simulink model "linear_exp_2025a"  (R2025a)
settings: Solver=FixedStepDiscrete  StartTime=0.0  StopTime=Inf  FixedStep=Ts  RelTol=1e-3
model workspace (MAT data in the model file):
  p_active = Simulink.Parameter
  p_active.Value = 1
  p_active.Complexity = 'real'
  p_active.Dimensions = [1 1]
  p_active.DataType = 'auto'
  p_ff = Simulink.Parameter
  p_ff.Value = [-1.41559534854 -1.58206727697 -1.65093789551 -1.60998265668 -1.49289778237 -1.36268185504 -1.28204754292 -1.28521947357 -1.3635848216 -1.47038204607 -1.54100339838 -1.51955701219 ... (800000 elements, 1x800000)]
  p_ff.Complexity = 'real'
  p_ff.Dimensions = [1 800000]
  p_ff.DataType = 'auto'
  p_ref = Simulink.Parameter
  p_ref.Value = [0 0 0 0 0 0 0 0 0 0 0 0 ... (800000 elements, 800000x1)]
  p_ref.Complexity = 'real'
  p_ref.Dimensions = [800000 1]
  p_ref.DataType = 'auto'
  p_servo = Simulink.Parameter
  p_servo.Value = 0
  p_servo.Complexity = 'real'
  p_servo.Dimensions = [1 1]
  p_servo.DataType = 'auto'
  servo_switch = Simulink.Parameter
  servo_switch.Value = 1
  servo_switch.Complexity = 'real'
  servo_switch.Dimensions = [1 1]
  servo_switch.DataType = 'auto'
undefined symbols (not defined in the file): CURRENT_TO_UNIT, MAX_INPUT, N, PULSE_TO_WIDTH, TwinCAT, VELOCITY_RESOLUTION
libraries: TcTargetLib x5, dspsigops x2, cstblocks x1, simulink x1
settings Model: SimulationMode=external  Creator=AKZW  LastModifiedBy=AKZW
settings DataIOCC: SaveFormat=Array  ReturnWorkspaceOutputs=off
settings OptimizationCC: LocalBlockOutputs=off
settings DebuggingCC: InheritedTsInSrcMsg=none
settings SFSimCC: UsePrecompiledLibraries=Avoid
settings RTWCC: SystemTargetFile=TwinCatGrt.tlc  GenCodeOnly=on  GenerateMakefile=off  TemplateMakefile=tcgrt_msbuild.tmf  TargetLang=C++  Description=TwinCAT GRT Target
settings STFCustomTargetCC: SystemTargetFile=TwinCatGrt.tlc  TargetLangStandard=C++11 (ISO)  MultiwordLength=2048.0  DynamicStringBufferSize=256.0  ConcurrentExecutionCompliant=on  CombineOutputUpdateFcns=on  MatFileLogging=on  CPPClassGenCompliant=on  GRTInterface=off  TcCom_ExecutionInfoOutput=off  TcCom_OemLicenses=$<Project:OemLicenses>  TcCom_ModuleIcon=$<TE140x:Icon>  TcCom_AllowDataAreaForSharedData=off  TcProject_InstallPlcLibrary=off  TcProject_PublishParallel=on  TcCom_BlockIoDataAccess=Internal DataArea  TcProject_VersionSrc=$<LatestTMFile>  TcProject_ClassFactoryName=$<Project:Name>  TcPlcFb_OemLicenses=$<Project:OemLicenses>  TcPlcFb_UpdateExceptionHandling=CallerExceptions  TcCom_DataStoreReadOnly=off  TcCom_InputDataAccess=Input Destination DataArea  TcProject_PublishTcOSARMv8A=off  TcProject_DrvProductVersion=$<DrvFileVersion>  TcProject_ForceRebuildForPublish=off  TcCom_ExtModeRtAllowForParameterChange=on  TcProject_PublishTcUMx86=off  TcProject_PublishTcRTx64=on  TcProject_BuildSystem=Auto  TcProject_DataExchangeModulesVersion=$<ModuleGenerator:DataExchange:Version>  TcProject_UseDataExchangeModules=off  TcProject_Copyright=Copyright $<VendorName> $<LocalDateTime:%Y>  TcProject_Versioning=Versioned  TcCom_UpdateExceptionHandling=CallerExceptions  TcCom_ContStateDataAccess=Internal DataArea  TcProject_PublishPlatformtoolset=Auto  TcCom_OnlineChange=off  TcCom_ExtModeRtWaitForStart=on  TcCom_StepSizeAdaptation=RequireMatchingTaskCycleTime  TcCom_BlockIoReadOnly=on  TcCom_Legacy_ModuleBuildInfoParam=on  TcProject_PublishTcOSARMv7M=off  TcCom_ExtModeRtAllowExecutionCommands=on  TcCom_StrictAccessLock=on  TcCom_DataStoreCreateSymbols=on  TcCom_BlockDiagramDebugInfoExport=on  TcCom_BlockDiagramExport=on  TcProject_PublishTcUMx64=off  TcProject_PublishConfiguration=Release  TcCom_OriginalIoBlockNames=off  TcCom_InputCreateSymbols=on  TcProject_SignWithTwinCatCertificate=inherit default  TcCom_ExtendSignalResolution=off  TcCom_ModuleCaller=CyclicTask  TcProject_SignTwinCatCertName=TcTestCert  TcProject_StaticStlStringCapacity=Auto  TcProject_VendorIcon=$<TE140x:Icon>  TcCom_TcComWrapperFbPropertyMonitoring=NoMonitoring  TcProject_CLanguageStandard=Default  TcProject_UseNativeBlockDiagramExport=off  TcProject_CreateUniqueEnumItemNames=off  TcCom_MaxInternalDataAreaParts=5U  TcCom_GroupIcon=$<TE140x:Icon>  TcProject_ProductName=$<ModuleGenerator:ProductId> $<ModuleGenerator:Version:MAJOR.MINOR>  TcPlcFb_MonitorExecutionTime=off  TcCom_DataStoreDataAccess=None  TcCom_DWorkReadOnly=on  TcProject_BuildWithWdk=inherit default  TcProject_PreferIntOverLong=off  TcCom_BlockIoCreateSymbols=on  TcProject_Publish=on  TcProject_PreferToolArchitectureX64=on  TcProject_EnableNewPlatforms=off  TcProject_UseStaticStlString=off  TcCom_VariableSymbolMapping=Identical  TcCom_DWorkCreateSymbols=on  TcCom_BlockDiagramVariableAccess=AssignToParent  TcCom_GroupName=TE140x|Simulink Modules  TcCom_Generate=on  TcProject_PlcVarPrefixes=PVOID=p | BOOL=b | BOOL32=b | DATE=d | TIME_OF_DATE=td | TIME=t | LTIME=t | GUID=n  TcCom_InputReadOnly=off  TcProject_Generate=on  TcCom_CallerVerification=Default  TcProject_UseLLVMCodeInfo=on  TcCom_ExecuteModelCode=on  TcCom_OnlineChangeRestoreDataAreas=off  TcPlcFb_ExtModeRtWaitForStart=off  TcCom_ContStateCreateSymbols=on  TcCom_ParametersInitValues=on  TcProject_IgnorePseudoArrayDimensions=off  TcProject_MaxVisibleArrayElements=200U  TcCom_DWorkDataAccess=Internal DataArea  TcCom_ResolveMaskedSubsystems=off  TcProject_GenerateVsSolution=No  TcProject_UseIntrinsics=on  TcCom_OutputCreateSymbols=on  TcCom_ExecutionSequence=UpdateBeforeOutputMapping  TcProject_UseCodeDescriptor=on  TcCom_GroupDisplayName=$<GroupName>  TcProject_Description=TwinCAT executable file, generated by TwinCAT $<ModuleGenerator:ProductId>  TcPlcFb_ExtModeRtAllowForParameterChange=off  TcCom_ParametersCreateSymbols=on  TcCom_AccessLockState=Auto  TcProject_DeployRestart=off  TcProject_PublishTcOSARMv7A=off  TcProject_CppLanguageStandard=Default  TcProject_UseDescriptorCodeType=on  TcPlcFb_ExtModeRtAllowExecutionCommands=off  TcCom_GlobalParamDefaultSharing=Define  TcCom_OutputDataAccess=Output Source DataArea  TcProject_PublishTcOSx64E=off  TcProject_CreateScopedEnums=Auto  TcProject_IncrementVersion=Revision  TcCom_TcComWrapperFb=off  TcProject_Verbosity=Normal  TcProject_DrvFileVersion=$<VersionFromFile>  TcCom_TcComWrapperFbProperties=off  TcProject_GeneratePlcLibrary=off  TcProject_PublishTcRTx86=on  TcPlcFb_InitExceptionHandling=CallerExceptions  TcPlcFb_Generate=off  TcCom_ContStateReadOnly=on  TcCom_ParametersReadOnly=off  TcCom_ExecutionInfoParam=on  TcCom_OutputReadOnly=on  TcCom_MonitorExecutionTime=off  TcProject_LibraryCategories=$<VendorName>  TcProject_LowestCompatibleTcBuild=$<TwinCAT:Version:BUILD>  TcCom_ParametersDataAccess=Internal DataArea  TcProject_GenerateStructDutsWithDefaultValues=Auto  TcProject_UseTmxExtension=Auto  TcCom_InputInitValues=off  TcProject_LibCatPath=$<Project:Dir>\$<Project:Name>.libcat.xml  TcProject_VendorName=TE140x Module Vendor  TcCom_InitExceptionHandling=CallerExceptions  TcProject_TmxInstall=on  TcProject_PublishTcOSx64=off  TcCom_VariableSymbolMappingCustom=$<ModelName>_U=Input|$<ModelName>_Y=Output|$<ModelName>_P=ModelParameters|$<ModelName>_B=BlockIO|$<ModelName>_DW=DWork|$<ModelName>_X=ContStates  TcProject_UseCodeInfoExporter=on  TcProject_CoderCppNamespace=coder
settings GRTTargetCC: ExtMode=on  ExtModeMexFile=TcExtModeClient  TargetLangStandard=C++11 (ISO)  ParMdlRefBuildCompliant=off  CompOptLevelCompliant=off  UseToolchainInfoCompliant=off

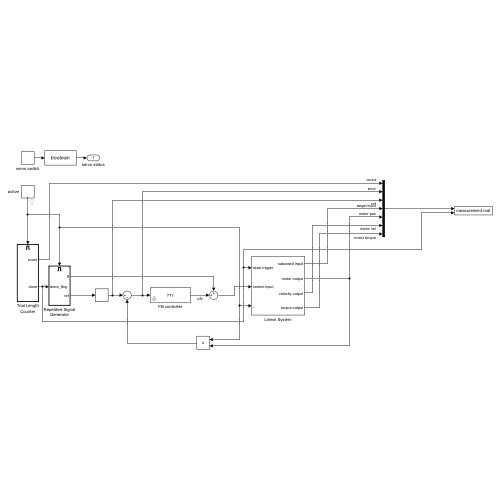
[thumbnail: Simulink's stored preview of the top-level diagram]
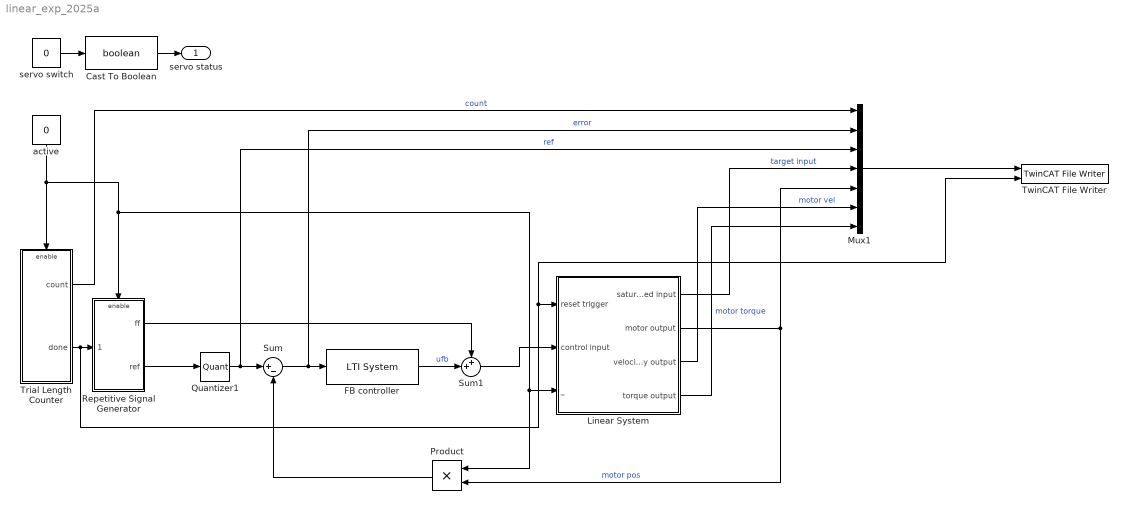
== system linear_exp_2025a ==
  Cast To Boolean : DataTypeConversion  OutDataTypeStr=boolean  SaturateOnIntegerOverflow=off  RndMeth=Floor
  FB controller : cstblocks/LTI System  sys=Kd  IC=[]  PadeOrder=0
  Linear System : Subsystem
  Mux1 : Mux  Inputs=7
  Product : Product
  Quantizer1 : Quantizer  QuantizationInterval=ENCODER_RESOLUTION
  Repetitive Signal Generator : Subsystem
  Sum : Sum  Inputs=|+-
  Sum1 : Sum  Inputs=++|
  Trial Length Counter : Subsystem
  TwinCAT File Writer : TcTargetLib/TwinCAT File Writer  PortDataType=Inherit: auto  PortDim=-1  SampleTime=-1  MatFileName=C:\expdata\measurement.mat  MaxFileByteSize=0  MaxFileCount=0  Pause=on  TraceMode=3  WriteTimestamp=on  PauseAsInput=on  CloseOnPause=on
      settings: SourceProductName=Beckhoff TwinCAT Target
  active : Constant  Value=0
  servo switch : Constant  Value=0
  servo status : Outport  VectorParamsAs1DForOutWhenUnconnected=off
  wires:
  active/1 -> Trial Length Counter/Enable, Repetitive Signal Generator/Enable, Product/1, Linear System/3(_)
  Product/1 -> Sum/2
  Repetitive Signal Generator/1(ff) -> Sum1/1
  Linear System/2(motor output) -> Mux1/5, Product/2  "motor pos"
  Mux1/1 -> TwinCAT File Writer/1
  Quantizer1/1 -> Mux1/3, Sum/1  "ref"
  Linear System/4(torque output) -> Mux1/7  "motor torque"
  Sum/1 -> Mux1/2, FB controller/1  "error"
  Linear System/3(velocity output) -> Mux1/6  "motor vel"
  Cast To Boolean/1 -> servo status/1
  Trial Length Counter/1(count) -> Mux1/1  "count"
  Trial Length Counter/2(done) -> TwinCAT File Writer/2, Linear System/1(reset trigger), Repetitive Signal Generator/1(done_flag)
  FB controller/1 -> Sum1/2  "ufb"
  servo switch/1 -> Cast To Boolean/1
  Repetitive Signal Generator/2(ref) -> Quantizer1/1
  Sum1/1 -> Linear System/2(control input)
  Linear System/1(saturated input) -> Mux1/4  "target input"

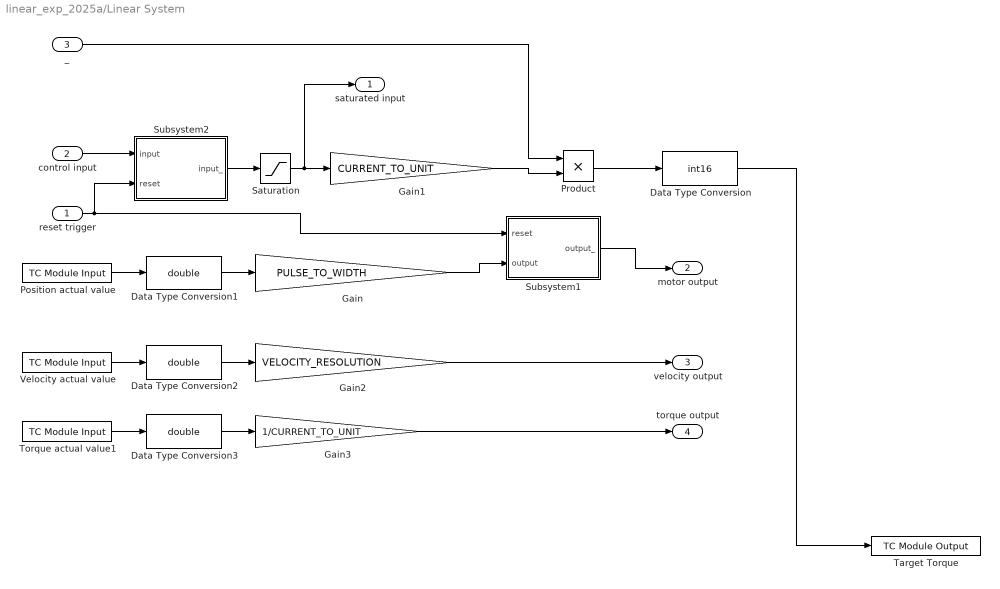
== system linear_exp_2025a/Linear System ==
  reset trigger : Inport
  control input : Inport  Port=2
  _ : Inport  Port=3
  " Torque actual value1" : TcTargetLib/TC Module Input  PortDataType=int16  Value=0  SampleTime=-1  PortDim=-1  PortComplexity=auto  SymbolName=TwinCAT.ModuleGenerator.Simulink.BlockPathToSymbolName(gcb,true)  CodeGenConnectType=DataArea (InputDst)  DataTypeOverride=off
      settings: SourceProductName=Beckhoff TwinCAT Target
  " Velocity actual value" : TcTargetLib/TC Module Input  PortDataType=int32  Value=0  SampleTime=-1  PortDim=-1  PortComplexity=auto  SymbolName=TwinCAT.ModuleGenerator.Simulink.BlockPathToSymbolName(gcb,true)  CodeGenConnectType=DataArea (InputDst)  DataTypeOverride=off
      settings: SourceProductName=Beckhoff TwinCAT Target
  Data Type Conversion : DataTypeConversion  OutDataTypeStr=int16  SaturateOnIntegerOverflow=off  RndMeth=Floor
  Data Type Conversion1 : DataTypeConversion  OutDataTypeStr=double  SaturateOnIntegerOverflow=off  RndMeth=Floor
  Data Type Conversion2 : DataTypeConversion  OutDataTypeStr=double  SaturateOnIntegerOverflow=off  RndMeth=Floor
  Data Type Conversion3 : DataTypeConversion  OutDataTypeStr=double  SaturateOnIntegerOverflow=off  RndMeth=Floor
  Gain : Gain  Gain=PULSE_TO_WIDTH
  Gain1 : Gain  Gain=CURRENT_TO_UNIT
  Gain2 : Gain  Gain=VELOCITY_RESOLUTION
  Gain3 : Gain  Gain=1/CURRENT_TO_UNIT
  Position actual value : TcTargetLib/TC Module Input  PortDataType=int32  Value=0  SampleTime=-1  PortDim=-1  PortComplexity=auto  SymbolName=TwinCAT.ModuleGenerator.Simulink.BlockPathToSymbolName(gcb,true)  CodeGenConnectType=DataArea (InputDst)  DataTypeOverride=off
      settings: SourceProductName=Beckhoff TwinCAT Target
  Product : Product
  Saturation : Saturate  UpperLimit=MAX_INPUT  LowerLimit=-MAX_INPUT
  Subsystem1 : Subsystem
  Subsystem2 : Subsystem
  Target Torque : TcTargetLib/TC Module Output  PortDataType=int16  SampleTime=-1  PortDim=-1  PortComplexity=auto  SymbolName=TwinCAT.ModuleGenerator.Simulink.BlockPathToSymbolName(gcb,true)  CodeGenConnectType=DataArea (OutputSrc)  DataTypeOverride=off
      settings: SourceProductName=Beckhoff TwinCAT Target
  saturated input : Outport  VectorParamsAs1DForOutWhenUnconnected=off
  motor output : Outport  Port=2  VectorParamsAs1DForOutWhenUnconnected=off
  velocity output : Outport  Port=3  VectorParamsAs1DForOutWhenUnconnected=off
  torque output : Outport  Port=4  VectorParamsAs1DForOutWhenUnconnected=off
  wires:
  Data Type Conversion1/1 -> Gain/1
  Gain/1 -> Subsystem1/2(output)
  Position actual value/1 -> Data Type Conversion1/1
  control input/1 -> Subsystem2/1(input)
  Subsystem1/1(output_) -> motor output/1
  Subsystem2/1(input_) -> Saturation/1
  Saturation/1 -> saturated input/1, Gain1/1
  reset trigger/1 -> Subsystem1/1(reset), Subsystem2/2(reset)
  Data Type Conversion2/1 -> Gain2/1
  " Velocity actual value"/1 -> Data Type Conversion2/1
  Gain2/1 -> velocity output/1
  " Torque actual value1"/1 -> Data Type Conversion3/1
  Data Type Conversion3/1 -> Gain3/1
  Gain3/1 -> torque output/1
  _/1 -> Product/1
  Gain1/1 -> Product/2
  Product/1 -> Data Type Conversion/1
  Data Type Conversion/1 -> Target Torque/1

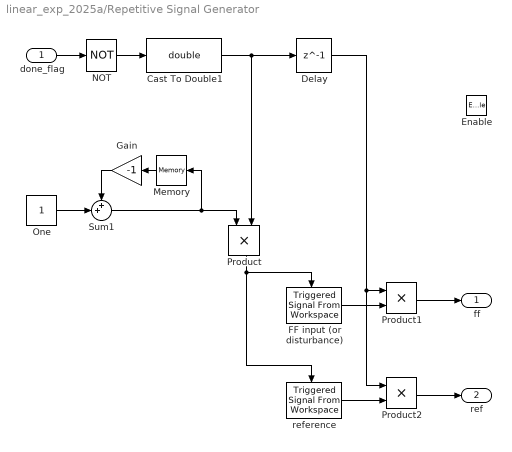
== system linear_exp_2025a/Repetitive Signal Generator ==
  done_flag : Inport
  Enable : EnablePort  StatesWhenEnabling=reset
  Cast To Double1 : DataTypeConversion  OutDataTypeStr=double  SaturateOnIntegerOverflow=off  RndMeth=Floor
  Delay : Delay  DelayLength=1
  "FF input (or disturbance) " : dspsigops/Triggered Signal From Workspace  Signal=set_ff  TriggerType=Either edge  ic=0  SamplesPerFrame=1  OutputAfterFinalValue=Cyclic repetition  OutputFrames=off
  Gain : Gain  Gain=-1
  Memory : Memory
  NOT : Logic  Operator=NOT  IconShape=distinctive  AllPortsSameDT=off  OutDataTypeStr=boolean
  One : Constant  OutDataTypeStr=Inherit: Inherit via back propagation
  Product : Product
  Product1 : Product
  Product2 : Product
  Sum1 : Sum  Inputs=++|
  reference : dspsigops/Triggered Signal From Workspace  Signal=set_ref  TriggerType=Either edge  ic=0  SamplesPerFrame=1  OutputAfterFinalValue=Cyclic repetition  OutputFrames=off
  ff : Outport  OutputWhenDisabled=reset  InitialOutput=0
  ref : Outport  Port=2  OutputWhenDisabled=reset  InitialOutput=0
  wires:
  "FF input (or disturbance) "/1 -> Product1/2
  Product1/1 -> ff/1
  Product/1 -> "FF input (or disturbance) "/Trigger, reference/Trigger
  Sum1/1 -> Product/1, Memory/1
  Gain/1 -> Sum1/1
  Memory/1 -> Gain/1
  One/1 -> Sum1/2
  done_flag/1 -> NOT/1
  Delay/1 -> Product1/1, Product2/1
  Product2/1 -> ref/1
  reference/1 -> Product2/2
  NOT/1 -> Cast To Double1/1
  Cast To Double1/1 -> Delay/1, Product/2

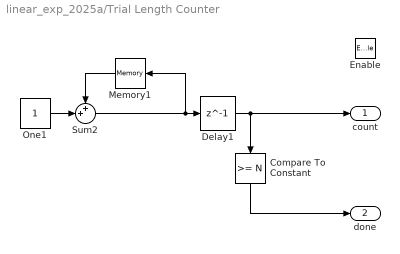
== system linear_exp_2025a/Trial Length Counter ==
  Enable : EnablePort  StatesWhenEnabling=reset
  Compare To Constant : simulink/Logic and Bit Operations/Compare To Constant  relop=>=  const=N  OutDataTypeStr=boolean
  Delay1 : Delay  DelayLength=1
  Memory1 : Memory
  One1 : Constant  OutDataTypeStr=Inherit: Inherit via back propagation
  Sum2 : Sum  Inputs=++|
  count : Outport  OutputWhenDisabled=reset  InitialOutput=0
  done : Outport  Port=2  InitialOutput=1
  wires:
  One1/1 -> Sum2/2
  Sum2/1 -> Delay1/1, Memory1/1
  Memory1/1 -> Sum2/1
  Delay1/1 -> count/1, Compare To Constant/1
  Compare To Constant/1 -> done/1

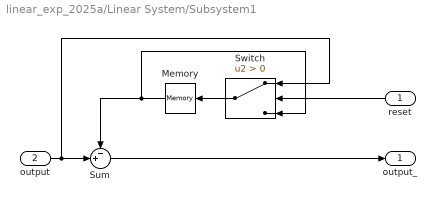
== system linear_exp_2025a/Linear System/Subsystem1 ==
  reset : Inport
  output : Inport  Port=2
  Memory : Memory
  Sum : Sum  Inputs=-+|
  Switch : Switch  Criteria=u2 > Threshold  SaturateOnIntegerOverflow=off  InputSameDT=off
  output_ : Outport  VectorParamsAs1DForOutWhenUnconnected=off
  wires:
  reset/1 -> Switch/2
  Sum/1 -> output_/1
  output/1 -> Sum/2, Switch/1
  Switch/1 -> Memory/1
  Memory/1 -> Sum/1, Switch/3

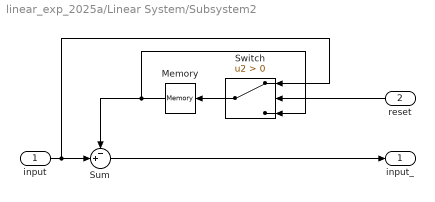
== system linear_exp_2025a/Linear System/Subsystem2 ==
  input : Inport
  reset : Inport  Port=2
  Memory : Memory
  Sum : Sum  Inputs=-+|
  Switch : Switch  Criteria=u2 > Threshold  SaturateOnIntegerOverflow=off  InputSameDT=off
  input_ : Outport  VectorParamsAs1DForOutWhenUnconnected=off
  wires:
  Memory/1 -> Switch/3, Sum/1
  Switch/1 -> Memory/1
  input/1 -> Switch/1, Sum/2
  Sum/1 -> input_/1
  reset/1 -> Switch/2
